simulink library "BatteryPack_v2"  (R2024b)
settings: Solver=VariableStepAuto  StartTime=0.0  StopTime=10.0  RelTol=1e-3
undefined symbols (not defined in the file or in its folder): battery_builder_rtmsupport, gcbh
libraries: BatteryPack_v2_lib x161
(part 6 of 8)

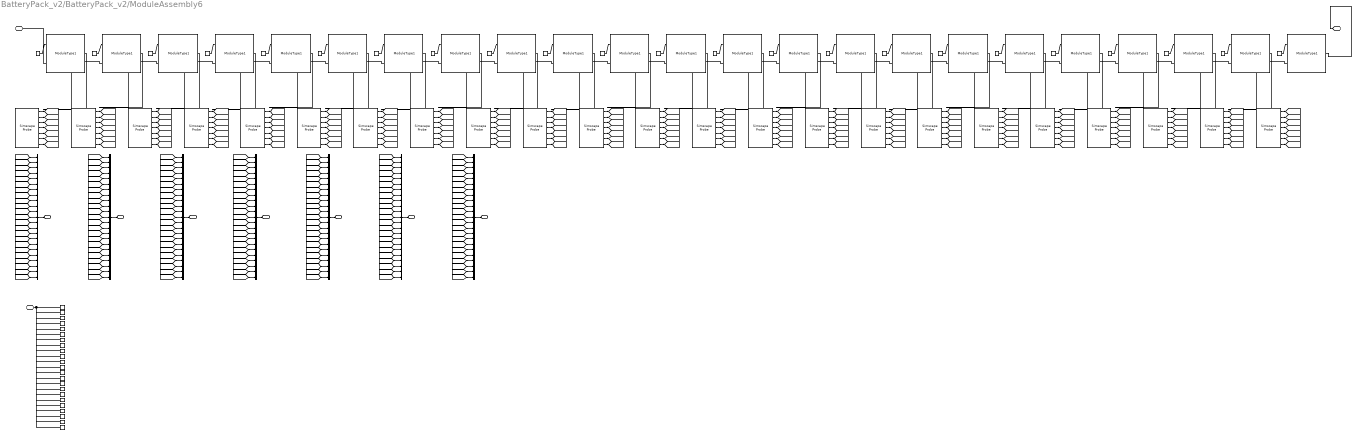
== system BatteryPack_v2/BatteryPack_v2/ModuleAssembly6 ==
  note: Thermal Boundary Conditions
  note: Output Signals
  note: Battery Modules
  AmbH_From_1 : ConnectionLabel  Label=ambH_1
  AmbH_From_10 : ConnectionLabel  Label=ambH_10
  AmbH_From_11 : ConnectionLabel  Label=ambH_11
  AmbH_From_12 : ConnectionLabel  Label=ambH_12
  AmbH_From_13 : ConnectionLabel  Label=ambH_13
  AmbH_From_14 : ConnectionLabel  Label=ambH_14
  AmbH_From_15 : ConnectionLabel  Label=ambH_15
  AmbH_From_16 : ConnectionLabel  Label=ambH_16
  AmbH_From_17 : ConnectionLabel  Label=ambH_17
  AmbH_From_18 : ConnectionLabel  Label=ambH_18
  AmbH_From_19 : ConnectionLabel  Label=ambH_19
  AmbH_From_2 : ConnectionLabel  Label=ambH_2
  AmbH_From_20 : ConnectionLabel  Label=ambH_20
  AmbH_From_21 : ConnectionLabel  Label=ambH_21
  AmbH_From_22 : ConnectionLabel  Label=ambH_22
  AmbH_From_23 : ConnectionLabel  Label=ambH_23
  AmbH_From_3 : ConnectionLabel  Label=ambH_3
  AmbH_From_4 : ConnectionLabel  Label=ambH_4
  AmbH_From_5 : ConnectionLabel  Label=ambH_5
  AmbH_From_6 : ConnectionLabel  Label=ambH_6
  AmbH_From_7 : ConnectionLabel  Label=ambH_7
  AmbH_From_8 : ConnectionLabel  Label=ambH_8
  AmbH_From_9 : ConnectionLabel  Label=ambH_9
  AmbH_To_1 : ConnectionLabel  Label=ambH_1
  AmbH_To_10 : ConnectionLabel  Label=ambH_10
  AmbH_To_11 : ConnectionLabel  Label=ambH_11
  AmbH_To_12 : ConnectionLabel  Label=ambH_12
  AmbH_To_13 : ConnectionLabel  Label=ambH_13
  AmbH_To_14 : ConnectionLabel  Label=ambH_14
  AmbH_To_15 : ConnectionLabel  Label=ambH_15
  AmbH_To_16 : ConnectionLabel  Label=ambH_16
  AmbH_To_17 : ConnectionLabel  Label=ambH_17
  AmbH_To_18 : ConnectionLabel  Label=ambH_18
  AmbH_To_19 : ConnectionLabel  Label=ambH_19
  AmbH_To_2 : ConnectionLabel  Label=ambH_2
  AmbH_To_20 : ConnectionLabel  Label=ambH_20
  AmbH_To_21 : ConnectionLabel  Label=ambH_21
  AmbH_To_22 : ConnectionLabel  Label=ambH_22
  AmbH_To_23 : ConnectionLabel  Label=ambH_23
  AmbH_To_3 : ConnectionLabel  Label=ambH_3
  AmbH_To_4 : ConnectionLabel  Label=ambH_4
  AmbH_To_5 : ConnectionLabel  Label=ambH_5
  AmbH_To_6 : ConnectionLabel  Label=ambH_6
  AmbH_To_7 : ConnectionLabel  Label=ambH_7
  AmbH_To_8 : ConnectionLabel  Label=ambH_8
  AmbH_To_9 : ConnectionLabel  Label=ambH_9
  Module02 : BatteryPack_v2_lib/Modules/ModuleType1  SOC_vecCell=[0, .1, .25, .5, .75, .9, 1]  T_vecCell=[278, 293, 313] K  V0_matCell=[3.49, 3.5, 3.51; 3.55, 3.57, 3.56; 3.62, 3.63, 3.64; 3.71, 3.71, 3.72; 3.91, 3.93, 3.94; 4.07, 4.08, 4.08; 4.19, 4.19, 4.19] V  V_rangeCell=[0, inf] V  R0_matCell=[.0117, .0085, .009; .011, .0085, .009; .0114, .0087, .0092; .0107, .0082, .0088; .0107, .0083, .0091; .0113, .0085, .0089; .0116, .0085, .0089] Ohm  AHCell=27 A*hr  extrapolation_optionCell=simscape.enum.extrapolation.nearest  N0Cell=100  dV0Cell=0  dR0Cell=0  dAHCell=0  thermal_massCell=100 J/K  AmbientResistance=25 K/W  P=1  S=1  iCell_specify=off  iCell_priority=None  iCell=0 A  iCell_nominal_specify=off  iCell_nominal_value=1  iCell_nominal_unit=A  vCell_specify=off  vCell_priority=None  vCell=0 V  vCell_nominal_specify=off  vCell_nominal_value=1  vCell_nominal_unit=V  socCell_specify=off  socCell_priority=High  socCell=1  socCell_nominal_specify=off  socCell_nominal_value=1  socCell_nominal_unit=1  numCyclesCell_specify=off  numCyclesCell_priority=High  numCyclesCell=0  numCyclesCell_nominal_specify=off  numCyclesCell_nominal_value=1  numCyclesCell_nominal_unit=1  temperatureCell_specify=off  temperatureCell_priority=High  temperatureCell=298.15 K  temperatureCell_nominal_specify=off  temperatureCell_nominal_value=1  temperatureCell_nominal_unit=K  vParallelAssembly_specify=off  vParallelAssembly_priority=None  vParallelAssembly=0 V  vParallelAssembly_nominal_specify=off  vParallelAssembly_nominal_value=1  vParallelAssembly_nominal_unit=V  socParallelAssembly_specify=off  socParallelAssembly_priority=None  socParallelAssembly=1  socParallelAssembly_nominal_specify=off  socParallelAssembly_nominal_value=1  socParallelAssembly_nominal_unit=1
      settings: InternalSimscapePortConfiguration="{\"Bottom\":[{\"id\":\"n\",\"label\":\"-\",\"type\":\"foundation.electrical.electrical\"}],\"Left\":[{\"id\":\"AmbH\",\"label\":\"AmbH\",\"type\":\"foundation.thermal.thermal\"}],\"Right\":[],\"Top\":[{\"id\":\"p\",\"label\":\"+\",\"type\":\"foundation.electrical.electrical\"}]}"
  Module02_outputs : SimscapeProbe  BoundBlock=2660  Variables="{\"iCell\":{\"Unit\":\"A\",\"PortLabel\":\"iCell\",\"Probing\":\"ON\"},\"numCyclesCell\":{\"Unit\":\"1\",\"PortLabel\":\"numCyclesCell\",\"Probing\":\"ON\"},\"socCell\":{\"Unit\":\"1\",\"PortLabel\":\"socCell\",\"Probing\":\"ON\"},\"socParallelAssembly\":{\"Unit\":\"1\",\"PortLabel\":\"socParallelAssembly\",\"Probing\":\"ON\"},\"temperatureCell\":{\"Unit\":\"K\",\"PortLabel\":\"temperatureCell\",\"Probing\":\"ON\"},\"vCell\":{\"Unit\":\"V\",\"PortLabel\":\"vCell\",\"Probing\":\"ON\"},\"vParallelAssembly\":{\"Unit\":\"V\",\"PortLabel\":\"vParallelAssembly\",\"Probing\":\"ON\"}}"
  Module03 : BatteryPack_v2_lib/Modules/ModuleType1  SOC_vecCell=[0, .1, .25, .5, .75, .9, 1]  T_vecCell=[278, 293, 313] K  V0_matCell=[3.49, 3.5, 3.51; 3.55, 3.57, 3.56; 3.62, 3.63, 3.64; 3.71, 3.71, 3.72; 3.91, 3.93, 3.94; 4.07, 4.08, 4.08; 4.19, 4.19, 4.19] V  V_rangeCell=[0, inf] V  R0_matCell=[.0117, .0085, .009; .011, .0085, .009; .0114, .0087, .0092; .0107, .0082, .0088; .0107, .0083, .0091; .0113, .0085, .0089; .0116, .0085, .0089] Ohm  AHCell=27 A*hr  extrapolation_optionCell=simscape.enum.extrapolation.nearest  N0Cell=100  dV0Cell=0  dR0Cell=0  dAHCell=0  thermal_massCell=100 J/K  AmbientResistance=25 K/W  P=1  S=1  iCell_specify=off  iCell_priority=None  iCell=0 A  iCell_nominal_specify=off  iCell_nominal_value=1  iCell_nominal_unit=A  vCell_specify=off  vCell_priority=None  vCell=0 V  vCell_nominal_specify=off  vCell_nominal_value=1  vCell_nominal_unit=V  socCell_specify=off  socCell_priority=High  socCell=1  socCell_nominal_specify=off  socCell_nominal_value=1  socCell_nominal_unit=1  numCyclesCell_specify=off  numCyclesCell_priority=High  numCyclesCell=0  numCyclesCell_nominal_specify=off  numCyclesCell_nominal_value=1  numCyclesCell_nominal_unit=1  temperatureCell_specify=off  temperatureCell_priority=High  temperatureCell=298.15 K  temperatureCell_nominal_specify=off  temperatureCell_nominal_value=1  temperatureCell_nominal_unit=K  vParallelAssembly_specify=off  vParallelAssembly_priority=None  vParallelAssembly=0 V  vParallelAssembly_nominal_specify=off  vParallelAssembly_nominal_value=1  vParallelAssembly_nominal_unit=V  socParallelAssembly_specify=off  socParallelAssembly_priority=None  socParallelAssembly=1  socParallelAssembly_nominal_specify=off  socParallelAssembly_nominal_value=1  socParallelAssembly_nominal_unit=1
      settings: InternalSimscapePortConfiguration="{\"Bottom\":[{\"id\":\"n\",\"label\":\"-\",\"type\":\"foundation.electrical.electrical\"}],\"Left\":[{\"id\":\"AmbH\",\"label\":\"AmbH\",\"type\":\"foundation.thermal.thermal\"}],\"Right\":[],\"Top\":[{\"id\":\"p\",\"label\":\"+\",\"type\":\"foundation.electrical.electrical\"}]}"
  Module03_outputs : SimscapeProbe  BoundBlock=2662  Variables="{\"iCell\":{\"Unit\":\"A\",\"PortLabel\":\"iCell\",\"Probing\":\"ON\"},\"numCyclesCell\":{\"Unit\":\"1\",\"PortLabel\":\"numCyclesCell\",\"Probing\":\"ON\"},\"socCell\":{\"Unit\":\"1\",\"PortLabel\":\"socCell\",\"Probing\":\"ON\"},\"socParallelAssembly\":{\"Unit\":\"1\",\"PortLabel\":\"socParallelAssembly\",\"Probing\":\"ON\"},\"temperatureCell\":{\"Unit\":\"K\",\"PortLabel\":\"temperatureCell\",\"Probing\":\"ON\"},\"vCell\":{\"Unit\":\"V\",\"PortLabel\":\"vCell\",\"Probing\":\"ON\"},\"vParallelAssembly\":{\"Unit\":\"V\",\"PortLabel\":\"vParallelAssembly\",\"Probing\":\"ON\"}}"
  Module04 : BatteryPack_v2_lib/Modules/ModuleType1  SOC_vecCell=[0, .1, .25, .5, .75, .9, 1]  T_vecCell=[278, 293, 313] K  V0_matCell=[3.49, 3.5, 3.51; 3.55, 3.57, 3.56; 3.62, 3.63, 3.64; 3.71, 3.71, 3.72; 3.91, 3.93, 3.94; 4.07, 4.08, 4.08; 4.19, 4.19, 4.19] V  V_rangeCell=[0, inf] V  R0_matCell=[.0117, .0085, .009; .011, .0085, .009; .0114, .0087, .0092; .0107, .0082, .0088; .0107, .0083, .0091; .0113, .0085, .0089; .0116, .0085, .0089] Ohm  AHCell=27 A*hr  extrapolation_optionCell=simscape.enum.extrapolation.nearest  N0Cell=100  dV0Cell=0  dR0Cell=0  dAHCell=0  thermal_massCell=100 J/K  AmbientResistance=25 K/W  P=1  S=1  iCell_specify=off  iCell_priority=None  iCell=0 A  iCell_nominal_specify=off  iCell_nominal_value=1  iCell_nominal_unit=A  vCell_specify=off  vCell_priority=None  vCell=0 V  vCell_nominal_specify=off  vCell_nominal_value=1  vCell_nominal_unit=V  socCell_specify=off  socCell_priority=High  socCell=1  socCell_nominal_specify=off  socCell_nominal_value=1  socCell_nominal_unit=1  numCyclesCell_specify=off  numCyclesCell_priority=High  numCyclesCell=0  numCyclesCell_nominal_specify=off  numCyclesCell_nominal_value=1  numCyclesCell_nominal_unit=1  temperatureCell_specify=off  temperatureCell_priority=High  temperatureCell=298.15 K  temperatureCell_nominal_specify=off  temperatureCell_nominal_value=1  temperatureCell_nominal_unit=K  vParallelAssembly_specify=off  vParallelAssembly_priority=None  vParallelAssembly=0 V  vParallelAssembly_nominal_specify=off  vParallelAssembly_nominal_value=1  vParallelAssembly_nominal_unit=V  socParallelAssembly_specify=off  socParallelAssembly_priority=None  socParallelAssembly=1  socParallelAssembly_nominal_specify=off  socParallelAssembly_nominal_value=1  socParallelAssembly_nominal_unit=1
      settings: InternalSimscapePortConfiguration="{\"Bottom\":[{\"id\":\"n\",\"label\":\"-\",\"type\":\"foundation.electrical.electrical\"}],\"Left\":[{\"id\":\"AmbH\",\"label\":\"AmbH\",\"type\":\"foundation.thermal.thermal\"}],\"Right\":[],\"Top\":[{\"id\":\"p\",\"label\":\"+\",\"type\":\"foundation.electrical.electrical\"}]}"
  Module04_outputs : SimscapeProbe  BoundBlock=2664  Variables="{\"iCell\":{\"Unit\":\"A\",\"PortLabel\":\"iCell\",\"Probing\":\"ON\"},\"numCyclesCell\":{\"Unit\":\"1\",\"PortLabel\":\"numCyclesCell\",\"Probing\":\"ON\"},\"socCell\":{\"Unit\":\"1\",\"PortLabel\":\"socCell\",\"Probing\":\"ON\"},\"socParallelAssembly\":{\"Unit\":\"1\",\"PortLabel\":\"socParallelAssembly\",\"Probing\":\"ON\"},\"temperatureCell\":{\"Unit\":\"K\",\"PortLabel\":\"temperatureCell\",\"Probing\":\"ON\"},\"vCell\":{\"Unit\":\"V\",\"PortLabel\":\"vCell\",\"Probing\":\"ON\"},\"vParallelAssembly\":{\"Unit\":\"V\",\"PortLabel\":\"vParallelAssembly\",\"Probing\":\"ON\"}}"
  Module05 : BatteryPack_v2_lib/Modules/ModuleType1  SOC_vecCell=[0, .1, .25, .5, .75, .9, 1]  T_vecCell=[278, 293, 313] K  V0_matCell=[3.49, 3.5, 3.51; 3.55, 3.57, 3.56; 3.62, 3.63, 3.64; 3.71, 3.71, 3.72; 3.91, 3.93, 3.94; 4.07, 4.08, 4.08; 4.19, 4.19, 4.19] V  V_rangeCell=[0, inf] V  R0_matCell=[.0117, .0085, .009; .011, .0085, .009; .0114, .0087, .0092; .0107, .0082, .0088; .0107, .0083, .0091; .0113, .0085, .0089; .0116, .0085, .0089] Ohm  AHCell=27 A*hr  extrapolation_optionCell=simscape.enum.extrapolation.nearest  N0Cell=100  dV0Cell=0  dR0Cell=0  dAHCell=0  thermal_massCell=100 J/K  AmbientResistance=25 K/W  P=1  S=1  iCell_specify=off  iCell_priority=None  iCell=0 A  iCell_nominal_specify=off  iCell_nominal_value=1  iCell_nominal_unit=A  vCell_specify=off  vCell_priority=None  vCell=0 V  vCell_nominal_specify=off  vCell_nominal_value=1  vCell_nominal_unit=V  socCell_specify=off  socCell_priority=High  socCell=1  socCell_nominal_specify=off  socCell_nominal_value=1  socCell_nominal_unit=1  numCyclesCell_specify=off  numCyclesCell_priority=High  numCyclesCell=0  numCyclesCell_nominal_specify=off  numCyclesCell_nominal_value=1  numCyclesCell_nominal_unit=1  temperatureCell_specify=off  temperatureCell_priority=High  temperatureCell=298.15 K  temperatureCell_nominal_specify=off  temperatureCell_nominal_value=1  temperatureCell_nominal_unit=K  vParallelAssembly_specify=off  vParallelAssembly_priority=None  vParallelAssembly=0 V  vParallelAssembly_nominal_specify=off  vParallelAssembly_nominal_value=1  vParallelAssembly_nominal_unit=V  socParallelAssembly_specify=off  socParallelAssembly_priority=None  socParallelAssembly=1  socParallelAssembly_nominal_specify=off  socParallelAssembly_nominal_value=1  socParallelAssembly_nominal_unit=1
      settings: InternalSimscapePortConfiguration="{\"Bottom\":[{\"id\":\"n\",\"label\":\"-\",\"type\":\"foundation.electrical.electrical\"}],\"Left\":[{\"id\":\"AmbH\",\"label\":\"AmbH\",\"type\":\"foundation.thermal.thermal\"}],\"Right\":[],\"Top\":[{\"id\":\"p\",\"label\":\"+\",\"type\":\"foundation.electrical.electrical\"}]}"
  Module05_outputs : SimscapeProbe  BoundBlock=2666  Variables="{\"iCell\":{\"Unit\":\"A\",\"PortLabel\":\"iCell\",\"Probing\":\"ON\"},\"numCyclesCell\":{\"Unit\":\"1\",\"PortLabel\":\"numCyclesCell\",\"Probing\":\"ON\"},\"socCell\":{\"Unit\":\"1\",\"PortLabel\":\"socCell\",\"Probing\":\"ON\"},\"socParallelAssembly\":{\"Unit\":\"1\",\"PortLabel\":\"socParallelAssembly\",\"Probing\":\"ON\"},\"temperatureCell\":{\"Unit\":\"K\",\"PortLabel\":\"temperatureCell\",\"Probing\":\"ON\"},\"vCell\":{\"Unit\":\"V\",\"PortLabel\":\"vCell\",\"Probing\":\"ON\"},\"vParallelAssembly\":{\"Unit\":\"V\",\"PortLabel\":\"vParallelAssembly\",\"Probing\":\"ON\"}}"
  Module06 : BatteryPack_v2_lib/Modules/ModuleType1  SOC_vecCell=[0, .1, .25, .5, .75, .9, 1]  T_vecCell=[278, 293, 313] K  V0_matCell=[3.49, 3.5, 3.51; 3.55, 3.57, 3.56; 3.62, 3.63, 3.64; 3.71, 3.71, 3.72; 3.91, 3.93, 3.94; 4.07, 4.08, 4.08; 4.19, 4.19, 4.19] V  V_rangeCell=[0, inf] V  R0_matCell=[.0117, .0085, .009; .011, .0085, .009; .0114, .0087, .0092; .0107, .0082, .0088; .0107, .0083, .0091; .0113, .0085, .0089; .0116, .0085, .0089] Ohm  AHCell=27 A*hr  extrapolation_optionCell=simscape.enum.extrapolation.nearest  N0Cell=100  dV0Cell=0  dR0Cell=0  dAHCell=0  thermal_massCell=100 J/K  AmbientResistance=25 K/W  P=1  S=1  iCell_specify=off  iCell_priority=None  iCell=0 A  iCell_nominal_specify=off  iCell_nominal_value=1  iCell_nominal_unit=A  vCell_specify=off  vCell_priority=None  vCell=0 V  vCell_nominal_specify=off  vCell_nominal_value=1  vCell_nominal_unit=V  socCell_specify=off  socCell_priority=High  socCell=1  socCell_nominal_specify=off  socCell_nominal_value=1  socCell_nominal_unit=1  numCyclesCell_specify=off  numCyclesCell_priority=High  numCyclesCell=0  numCyclesCell_nominal_specify=off  numCyclesCell_nominal_value=1  numCyclesCell_nominal_unit=1  temperatureCell_specify=off  temperatureCell_priority=High  temperatureCell=298.15 K  temperatureCell_nominal_specify=off  temperatureCell_nominal_value=1  temperatureCell_nominal_unit=K  vParallelAssembly_specify=off  vParallelAssembly_priority=None  vParallelAssembly=0 V  vParallelAssembly_nominal_specify=off  vParallelAssembly_nominal_value=1  vParallelAssembly_nominal_unit=V  socParallelAssembly_specify=off  socParallelAssembly_priority=None  socParallelAssembly=1  socParallelAssembly_nominal_specify=off  socParallelAssembly_nominal_value=1  socParallelAssembly_nominal_unit=1
      settings: InternalSimscapePortConfiguration="{\"Bottom\":[{\"id\":\"n\",\"label\":\"-\",\"type\":\"foundation.electrical.electrical\"}],\"Left\":[{\"id\":\"AmbH\",\"label\":\"AmbH\",\"type\":\"foundation.thermal.thermal\"}],\"Right\":[],\"Top\":[{\"id\":\"p\",\"label\":\"+\",\"type\":\"foundation.electrical.electrical\"}]}"
  Module06_outputs : SimscapeProbe  BoundBlock=2668  Variables="{\"iCell\":{\"Unit\":\"A\",\"PortLabel\":\"iCell\",\"Probing\":\"ON\"},\"numCyclesCell\":{\"Unit\":\"1\",\"PortLabel\":\"numCyclesCell\",\"Probing\":\"ON\"},\"socCell\":{\"Unit\":\"1\",\"PortLabel\":\"socCell\",\"Probing\":\"ON\"},\"socParallelAssembly\":{\"Unit\":\"1\",\"PortLabel\":\"socParallelAssembly\",\"Probing\":\"ON\"},\"temperatureCell\":{\"Unit\":\"K\",\"PortLabel\":\"temperatureCell\",\"Probing\":\"ON\"},\"vCell\":{\"Unit\":\"V\",\"PortLabel\":\"vCell\",\"Probing\":\"ON\"},\"vParallelAssembly\":{\"Unit\":\"V\",\"PortLabel\":\"vParallelAssembly\",\"Probing\":\"ON\"}}"
  Module07 : BatteryPack_v2_lib/Modules/ModuleType1  SOC_vecCell=[0, .1, .25, .5, .75, .9, 1]  T_vecCell=[278, 293, 313] K  V0_matCell=[3.49, 3.5, 3.51; 3.55, 3.57, 3.56; 3.62, 3.63, 3.64; 3.71, 3.71, 3.72; 3.91, 3.93, 3.94; 4.07, 4.08, 4.08; 4.19, 4.19, 4.19] V  V_rangeCell=[0, inf] V  R0_matCell=[.0117, .0085, .009; .011, .0085, .009; .0114, .0087, .0092; .0107, .0082, .0088; .0107, .0083, .0091; .0113, .0085, .0089; .0116, .0085, .0089] Ohm  AHCell=27 A*hr  extrapolation_optionCell=simscape.enum.extrapolation.nearest  N0Cell=100  dV0Cell=0  dR0Cell=0  dAHCell=0  thermal_massCell=100 J/K  AmbientResistance=25 K/W  P=1  S=1  iCell_specify=off  iCell_priority=None  iCell=0 A  iCell_nominal_specify=off  iCell_nominal_value=1  iCell_nominal_unit=A  vCell_specify=off  vCell_priority=None  vCell=0 V  vCell_nominal_specify=off  vCell_nominal_value=1  vCell_nominal_unit=V  socCell_specify=off  socCell_priority=High  socCell=1  socCell_nominal_specify=off  socCell_nominal_value=1  socCell_nominal_unit=1  numCyclesCell_specify=off  numCyclesCell_priority=High  numCyclesCell=0  numCyclesCell_nominal_specify=off  numCyclesCell_nominal_value=1  numCyclesCell_nominal_unit=1  temperatureCell_specify=off  temperatureCell_priority=High  temperatureCell=298.15 K  temperatureCell_nominal_specify=off  temperatureCell_nominal_value=1  temperatureCell_nominal_unit=K  vParallelAssembly_specify=off  vParallelAssembly_priority=None  vParallelAssembly=0 V  vParallelAssembly_nominal_specify=off  vParallelAssembly_nominal_value=1  vParallelAssembly_nominal_unit=V  socParallelAssembly_specify=off  socParallelAssembly_priority=None  socParallelAssembly=1  socParallelAssembly_nominal_specify=off  socParallelAssembly_nominal_value=1  socParallelAssembly_nominal_unit=1
      settings: InternalSimscapePortConfiguration="{\"Bottom\":[{\"id\":\"n\",\"label\":\"-\",\"type\":\"foundation.electrical.electrical\"}],\"Left\":[{\"id\":\"AmbH\",\"label\":\"AmbH\",\"type\":\"foundation.thermal.thermal\"}],\"Right\":[],\"Top\":[{\"id\":\"p\",\"label\":\"+\",\"type\":\"foundation.electrical.electrical\"}]}"
  Module07_outputs : SimscapeProbe  BoundBlock=2670  Variables="{\"iCell\":{\"Unit\":\"A\",\"PortLabel\":\"iCell\",\"Probing\":\"ON\"},\"numCyclesCell\":{\"Unit\":\"1\",\"PortLabel\":\"numCyclesCell\",\"Probing\":\"ON\"},\"socCell\":{\"Unit\":\"1\",\"PortLabel\":\"socCell\",\"Probing\":\"ON\"},\"socParallelAssembly\":{\"Unit\":\"1\",\"PortLabel\":\"socParallelAssembly\",\"Probing\":\"ON\"},\"temperatureCell\":{\"Unit\":\"K\",\"PortLabel\":\"temperatureCell\",\"Probing\":\"ON\"},\"vCell\":{\"Unit\":\"V\",\"PortLabel\":\"vCell\",\"Probing\":\"ON\"},\"vParallelAssembly\":{\"Unit\":\"V\",\"PortLabel\":\"vParallelAssembly\",\"Probing\":\"ON\"}}"
  Module08 : BatteryPack_v2_lib/Modules/ModuleType1  SOC_vecCell=[0, .1, .25, .5, .75, .9, 1]  T_vecCell=[278, 293, 313] K  V0_matCell=[3.49, 3.5, 3.51; 3.55, 3.57, 3.56; 3.62, 3.63, 3.64; 3.71, 3.71, 3.72; 3.91, 3.93, 3.94; 4.07, 4.08, 4.08; 4.19, 4.19, 4.19] V  V_rangeCell=[0, inf] V  R0_matCell=[.0117, .0085, .009; .011, .0085, .009; .0114, .0087, .0092; .0107, .0082, .0088; .0107, .0083, .0091; .0113, .0085, .0089; .0116, .0085, .0089] Ohm  AHCell=27 A*hr  extrapolation_optionCell=simscape.enum.extrapolation.nearest  N0Cell=100  dV0Cell=0  dR0Cell=0  dAHCell=0  thermal_massCell=100 J/K  AmbientResistance=25 K/W  P=1  S=1  iCell_specify=off  iCell_priority=None  iCell=0 A  iCell_nominal_specify=off  iCell_nominal_value=1  iCell_nominal_unit=A  vCell_specify=off  vCell_priority=None  vCell=0 V  vCell_nominal_specify=off  vCell_nominal_value=1  vCell_nominal_unit=V  socCell_specify=off  socCell_priority=High  socCell=1  socCell_nominal_specify=off  socCell_nominal_value=1  socCell_nominal_unit=1  numCyclesCell_specify=off  numCyclesCell_priority=High  numCyclesCell=0  numCyclesCell_nominal_specify=off  numCyclesCell_nominal_value=1  numCyclesCell_nominal_unit=1  temperatureCell_specify=off  temperatureCell_priority=High  temperatureCell=298.15 K  temperatureCell_nominal_specify=off  temperatureCell_nominal_value=1  temperatureCell_nominal_unit=K  vParallelAssembly_specify=off  vParallelAssembly_priority=None  vParallelAssembly=0 V  vParallelAssembly_nominal_specify=off  vParallelAssembly_nominal_value=1  vParallelAssembly_nominal_unit=V  socParallelAssembly_specify=off  socParallelAssembly_priority=None  socParallelAssembly=1  socParallelAssembly_nominal_specify=off  socParallelAssembly_nominal_value=1  socParallelAssembly_nominal_unit=1
      settings: InternalSimscapePortConfiguration="{\"Bottom\":[{\"id\":\"n\",\"label\":\"-\",\"type\":\"foundation.electrical.electrical\"}],\"Left\":[{\"id\":\"AmbH\",\"label\":\"AmbH\",\"type\":\"foundation.thermal.thermal\"}],\"Right\":[],\"Top\":[{\"id\":\"p\",\"label\":\"+\",\"type\":\"foundation.electrical.electrical\"}]}"
  Module08_outputs : SimscapeProbe  BoundBlock=2672  Variables="{\"iCell\":{\"Unit\":\"A\",\"PortLabel\":\"iCell\",\"Probing\":\"ON\"},\"numCyclesCell\":{\"Unit\":\"1\",\"PortLabel\":\"numCyclesCell\",\"Probing\":\"ON\"},\"socCell\":{\"Unit\":\"1\",\"PortLabel\":\"socCell\",\"Probing\":\"ON\"},\"socParallelAssembly\":{\"Unit\":\"1\",\"PortLabel\":\"socParallelAssembly\",\"Probing\":\"ON\"},\"temperatureCell\":{\"Unit\":\"K\",\"PortLabel\":\"temperatureCell\",\"Probing\":\"ON\"},\"vCell\":{\"Unit\":\"V\",\"PortLabel\":\"vCell\",\"Probing\":\"ON\"},\"vParallelAssembly\":{\"Unit\":\"V\",\"PortLabel\":\"vParallelAssembly\",\"Probing\":\"ON\"}}"
  Module09 : BatteryPack_v2_lib/Modules/ModuleType1  SOC_vecCell=[0, .1, .25, .5, .75, .9, 1]  T_vecCell=[278, 293, 313] K  V0_matCell=[3.49, 3.5, 3.51; 3.55, 3.57, 3.56; 3.62, 3.63, 3.64; 3.71, 3.71, 3.72; 3.91, 3.93, 3.94; 4.07, 4.08, 4.08; 4.19, 4.19, 4.19] V  V_rangeCell=[0, inf] V  R0_matCell=[.0117, .0085, .009; .011, .0085, .009; .0114, .0087, .0092; .0107, .0082, .0088; .0107, .0083, .0091; .0113, .0085, .0089; .0116, .0085, .0089] Ohm  AHCell=27 A*hr  extrapolation_optionCell=simscape.enum.extrapolation.nearest  N0Cell=100  dV0Cell=0  dR0Cell=0  dAHCell=0  thermal_massCell=100 J/K  AmbientResistance=25 K/W  P=1  S=1  iCell_specify=off  iCell_priority=None  iCell=0 A  iCell_nominal_specify=off  iCell_nominal_value=1  iCell_nominal_unit=A  vCell_specify=off  vCell_priority=None  vCell=0 V  vCell_nominal_specify=off  vCell_nominal_value=1  vCell_nominal_unit=V  socCell_specify=off  socCell_priority=High  socCell=1  socCell_nominal_specify=off  socCell_nominal_value=1  socCell_nominal_unit=1  numCyclesCell_specify=off  numCyclesCell_priority=High  numCyclesCell=0  numCyclesCell_nominal_specify=off  numCyclesCell_nominal_value=1  numCyclesCell_nominal_unit=1  temperatureCell_specify=off  temperatureCell_priority=High  temperatureCell=298.15 K  temperatureCell_nominal_specify=off  temperatureCell_nominal_value=1  temperatureCell_nominal_unit=K  vParallelAssembly_specify=off  vParallelAssembly_priority=None  vParallelAssembly=0 V  vParallelAssembly_nominal_specify=off  vParallelAssembly_nominal_value=1  vParallelAssembly_nominal_unit=V  socParallelAssembly_specify=off  socParallelAssembly_priority=None  socParallelAssembly=1  socParallelAssembly_nominal_specify=off  socParallelAssembly_nominal_value=1  socParallelAssembly_nominal_unit=1
      settings: InternalSimscapePortConfiguration="{\"Bottom\":[{\"id\":\"n\",\"label\":\"-\",\"type\":\"foundation.electrical.electrical\"}],\"Left\":[{\"id\":\"AmbH\",\"label\":\"AmbH\",\"type\":\"foundation.thermal.thermal\"}],\"Right\":[],\"Top\":[{\"id\":\"p\",\"label\":\"+\",\"type\":\"foundation.electrical.electrical\"}]}"
  Module09_outputs : SimscapeProbe  BoundBlock=2674  Variables="{\"iCell\":{\"Unit\":\"A\",\"PortLabel\":\"iCell\",\"Probing\":\"ON\"},\"numCyclesCell\":{\"Unit\":\"1\",\"PortLabel\":\"numCyclesCell\",\"Probing\":\"ON\"},\"socCell\":{\"Unit\":\"1\",\"PortLabel\":\"socCell\",\"Probing\":\"ON\"},\"socParallelAssembly\":{\"Unit\":\"1\",\"PortLabel\":\"socParallelAssembly\",\"Probing\":\"ON\"},\"temperatureCell\":{\"Unit\":\"K\",\"PortLabel\":\"temperatureCell\",\"Probing\":\"ON\"},\"vCell\":{\"Unit\":\"V\",\"PortLabel\":\"vCell\",\"Probing\":\"ON\"},\"vParallelAssembly\":{\"Unit\":\"V\",\"PortLabel\":\"vParallelAssembly\",\"Probing\":\"ON\"}}"
  Module{10..23} (14 alike) : BatteryPack_v2_lib/Modules/ModuleType1  SOC_vecCell=[0, .1, .25, .5, .75, .9, 1]  T_vecCell=[278, 293, 313] K  V0_matCell=[3.49, 3.5, 3.51; 3.55, 3.57, 3.56; 3.62, 3.63, 3.64; 3.71, 3.71, 3.72; 3.91, 3.93, 3.94; 4.07, 4.08, 4.08; 4.19, 4.19, 4.19] V  V_rangeCell=[0, inf] V  R0_matCell=[.0117, .0085, .009; .011, .0085, .009; .0114, .0087, .0092; .0107, .0082, .0088; .0107, .0083, .0091; .0113, .0085, .0089; .0116, .0085, .0089] Ohm  AHCell=27 A*hr  extrapolation_optionCell=simscape.enum.extrapolation.nearest  N0Cell=100  dV0Cell=0  dR0Cell=0  dAHCell=0  thermal_massCell=100 J/K  AmbientResistance=25 K/W  P=1  S=1  iCell_specify=off  iCell_priority=None  iCell=0 A  iCell_nominal_specify=off  iCell_nominal_value=1  iCell_nominal_unit=A  vCell_specify=off  vCell_priority=None  vCell=0 V  vCell_nominal_specify=off  vCell_nominal_value=1  vCell_nominal_unit=V  socCell_specify=off  socCell_priority=High  socCell=1  socCell_nominal_specify=off  socCell_nominal_value=1  socCell_nominal_unit=1  numCyclesCell_specify=off  numCyclesCell_priority=High  numCyclesCell=0  numCyclesCell_nominal_specify=off  numCyclesCell_nominal_value=1  numCyclesCell_nominal_unit=1  temperatureCell_specify=off  temperatureCell_priority=High  temperatureCell=298.15 K  temperatureCell_nominal_specify=off  temperatureCell_nominal_value=1  temperatureCell_nominal_unit=K  vParallelAssembly_specify=off  vParallelAssembly_priority=None  vParallelAssembly=0 V  vParallelAssembly_nominal_specify=off  vParallelAssembly_nominal_value=1  vParallelAssembly_nominal_unit=V  socParallelAssembly_specify=off  socParallelAssembly_priority=None  socParallelAssembly=1  socParallelAssembly_nominal_specify=off  socParallelAssembly_nominal_value=1  socParallelAssembly_nominal_unit=1
      settings: InternalSimscapePortConfiguration="{\"Bottom\":[{\"id\":\"n\",\"label\":\"-\",\"type\":\"foundation.electrical.electrical\"}],\"Left\":[{\"id\":\"AmbH\",\"label\":\"AmbH\",\"type\":\"foundation.thermal.thermal\"}],\"Right\":[],\"Top\":[{\"id\":\"p\",\"label\":\"+\",\"type\":\"foundation.electrical.electrical\"}]}"
  Module10_outputs : SimscapeProbe  BoundBlock=2676  Variables="{\"iCell\":{\"Unit\":\"A\",\"PortLabel\":\"iCell\",\"Probing\":\"ON\"},\"numCyclesCell\":{\"Unit\":\"1\",\"PortLabel\":\"numCyclesCell\",\"Probing\":\"ON\"},\"socCell\":{\"Unit\":\"1\",\"PortLabel\":\"socCell\",\"Probing\":\"ON\"},\"socParallelAssembly\":{\"Unit\":\"1\",\"PortLabel\":\"socParallelAssembly\",\"Probing\":\"ON\"},\"temperatureCell\":{\"Unit\":\"K\",\"PortLabel\":\"temperatureCell\",\"Probing\":\"ON\"},\"vCell\":{\"Unit\":\"V\",\"PortLabel\":\"vCell\",\"Probing\":\"ON\"},\"vParallelAssembly\":{\"Unit\":\"V\",\"PortLabel\":\"vParallelAssembly\",\"Probing\":\"ON\"}}"
  Module11_outputs : SimscapeProbe  BoundBlock=2678  Variables="{\"iCell\":{\"Unit\":\"A\",\"PortLabel\":\"iCell\",\"Probing\":\"ON\"},\"numCyclesCell\":{\"Unit\":\"1\",\"PortLabel\":\"numCyclesCell\",\"Probing\":\"ON\"},\"socCell\":{\"Unit\":\"1\",\"PortLabel\":\"socCell\",\"Probing\":\"ON\"},\"socParallelAssembly\":{\"Unit\":\"1\",\"PortLabel\":\"socParallelAssembly\",\"Probing\":\"ON\"},\"temperatureCell\":{\"Unit\":\"K\",\"PortLabel\":\"temperatureCell\",\"Probing\":\"ON\"},\"vCell\":{\"Unit\":\"V\",\"PortLabel\":\"vCell\",\"Probing\":\"ON\"},\"vParallelAssembly\":{\"Unit\":\"V\",\"PortLabel\":\"vParallelAssembly\",\"Probing\":\"ON\"}}"
  Module12_outputs : SimscapeProbe  BoundBlock=2680  Variables="{\"iCell\":{\"Unit\":\"A\",\"PortLabel\":\"iCell\",\"Probing\":\"ON\"},\"numCyclesCell\":{\"Unit\":\"1\",\"PortLabel\":\"numCyclesCell\",\"Probing\":\"ON\"},\"socCell\":{\"Unit\":\"1\",\"PortLabel\":\"socCell\",\"Probing\":\"ON\"},\"socParallelAssembly\":{\"Unit\":\"1\",\"PortLabel\":\"socParallelAssembly\",\"Probing\":\"ON\"},\"temperatureCell\":{\"Unit\":\"K\",\"PortLabel\":\"temperatureCell\",\"Probing\":\"ON\"},\"vCell\":{\"Unit\":\"V\",\"PortLabel\":\"vCell\",\"Probing\":\"ON\"},\"vParallelAssembly\":{\"Unit\":\"V\",\"PortLabel\":\"vParallelAssembly\",\"Probing\":\"ON\"}}"
  Module13_outputs : SimscapeProbe  BoundBlock=2682  Variables="{\"iCell\":{\"Unit\":\"A\",\"PortLabel\":\"iCell\",\"Probing\":\"ON\"},\"numCyclesCell\":{\"Unit\":\"1\",\"PortLabel\":\"numCyclesCell\",\"Probing\":\"ON\"},\"socCell\":{\"Unit\":\"1\",\"PortLabel\":\"socCell\",\"Probing\":\"ON\"},\"socParallelAssembly\":{\"Unit\":\"1\",\"PortLabel\":\"socParallelAssembly\",\"Probing\":\"ON\"},\"temperatureCell\":{\"Unit\":\"K\",\"PortLabel\":\"temperatureCell\",\"Probing\":\"ON\"},\"vCell\":{\"Unit\":\"V\",\"PortLabel\":\"vCell\",\"Probing\":\"ON\"},\"vParallelAssembly\":{\"Unit\":\"V\",\"PortLabel\":\"vParallelAssembly\",\"Probing\":\"ON\"}}"
  Module14_outputs : SimscapeProbe  BoundBlock=2684  Variables="{\"iCell\":{\"Unit\":\"A\",\"PortLabel\":\"iCell\",\"Probing\":\"ON\"},\"numCyclesCell\":{\"Unit\":\"1\",\"PortLabel\":\"numCyclesCell\",\"Probing\":\"ON\"},\"socCell\":{\"Unit\":\"1\",\"PortLabel\":\"socCell\",\"Probing\":\"ON\"},\"socParallelAssembly\":{\"Unit\":\"1\",\"PortLabel\":\"socParallelAssembly\",\"Probing\":\"ON\"},\"temperatureCell\":{\"Unit\":\"K\",\"PortLabel\":\"temperatureCell\",\"Probing\":\"ON\"},\"vCell\":{\"Unit\":\"V\",\"PortLabel\":\"vCell\",\"Probing\":\"ON\"},\"vParallelAssembly\":{\"Unit\":\"V\",\"PortLabel\":\"vParallelAssembly\",\"Probing\":\"ON\"}}"
  Module15_outputs : SimscapeProbe  BoundBlock=2686  Variables="{\"iCell\":{\"Unit\":\"A\",\"PortLabel\":\"iCell\",\"Probing\":\"ON\"},\"numCyclesCell\":{\"Unit\":\"1\",\"PortLabel\":\"numCyclesCell\",\"Probing\":\"ON\"},\"socCell\":{\"Unit\":\"1\",\"PortLabel\":\"socCell\",\"Probing\":\"ON\"},\"socParallelAssembly\":{\"Unit\":\"1\",\"PortLabel\":\"socParallelAssembly\",\"Probing\":\"ON\"},\"temperatureCell\":{\"Unit\":\"K\",\"PortLabel\":\"temperatureCell\",\"Probing\":\"ON\"},\"vCell\":{\"Unit\":\"V\",\"PortLabel\":\"vCell\",\"Probing\":\"ON\"},\"vParallelAssembly\":{\"Unit\":\"V\",\"PortLabel\":\"vParallelAssembly\",\"Probing\":\"ON\"}}"
  Module16_outputs : SimscapeProbe  BoundBlock=2688  Variables="{\"iCell\":{\"Unit\":\"A\",\"PortLabel\":\"iCell\",\"Probing\":\"ON\"},\"numCyclesCell\":{\"Unit\":\"1\",\"PortLabel\":\"numCyclesCell\",\"Probing\":\"ON\"},\"socCell\":{\"Unit\":\"1\",\"PortLabel\":\"socCell\",\"Probing\":\"ON\"},\"socParallelAssembly\":{\"Unit\":\"1\",\"PortLabel\":\"socParallelAssembly\",\"Probing\":\"ON\"},\"temperatureCell\":{\"Unit\":\"K\",\"PortLabel\":\"temperatureCell\",\"Probing\":\"ON\"},\"vCell\":{\"Unit\":\"V\",\"PortLabel\":\"vCell\",\"Probing\":\"ON\"},\"vParallelAssembly\":{\"Unit\":\"V\",\"PortLabel\":\"vParallelAssembly\",\"Probing\":\"ON\"}}"
  Module17_outputs : SimscapeProbe  BoundBlock=2690  Variables="{\"iCell\":{\"Unit\":\"A\",\"PortLabel\":\"iCell\",\"Probing\":\"ON\"},\"numCyclesCell\":{\"Unit\":\"1\",\"PortLabel\":\"numCyclesCell\",\"Probing\":\"ON\"},\"socCell\":{\"Unit\":\"1\",\"PortLabel\":\"socCell\",\"Probing\":\"ON\"},\"socParallelAssembly\":{\"Unit\":\"1\",\"PortLabel\":\"socParallelAssembly\",\"Probing\":\"ON\"},\"temperatureCell\":{\"Unit\":\"K\",\"PortLabel\":\"temperatureCell\",\"Probing\":\"ON\"},\"vCell\":{\"Unit\":\"V\",\"PortLabel\":\"vCell\",\"Probing\":\"ON\"},\"vParallelAssembly\":{\"Unit\":\"V\",\"PortLabel\":\"vParallelAssembly\",\"Probing\":\"ON\"}}"
  Module18_outputs : SimscapeProbe  BoundBlock=2692  Variables="{\"iCell\":{\"Unit\":\"A\",\"PortLabel\":\"iCell\",\"Probing\":\"ON\"},\"numCyclesCell\":{\"Unit\":\"1\",\"PortLabel\":\"numCyclesCell\",\"Probing\":\"ON\"},\"socCell\":{\"Unit\":\"1\",\"PortLabel\":\"socCell\",\"Probing\":\"ON\"},\"socParallelAssembly\":{\"Unit\":\"1\",\"PortLabel\":\"socParallelAssembly\",\"Probing\":\"ON\"},\"temperatureCell\":{\"Unit\":\"K\",\"PortLabel\":\"temperatureCell\",\"Probing\":\"ON\"},\"vCell\":{\"Unit\":\"V\",\"PortLabel\":\"vCell\",\"Probing\":\"ON\"},\"vParallelAssembly\":{\"Unit\":\"V\",\"PortLabel\":\"vParallelAssembly\",\"Probing\":\"ON\"}}"
  Module19_outputs : SimscapeProbe  BoundBlock=2694  Variables="{\"iCell\":{\"Unit\":\"A\",\"PortLabel\":\"iCell\",\"Probing\":\"ON\"},\"numCyclesCell\":{\"Unit\":\"1\",\"PortLabel\":\"numCyclesCell\",\"Probing\":\"ON\"},\"socCell\":{\"Unit\":\"1\",\"PortLabel\":\"socCell\",\"Probing\":\"ON\"},\"socParallelAssembly\":{\"Unit\":\"1\",\"PortLabel\":\"socParallelAssembly\",\"Probing\":\"ON\"},\"temperatureCell\":{\"Unit\":\"K\",\"PortLabel\":\"temperatureCell\",\"Probing\":\"ON\"},\"vCell\":{\"Unit\":\"V\",\"PortLabel\":\"vCell\",\"Probing\":\"ON\"},\"vParallelAssembly\":{\"Unit\":\"V\",\"PortLabel\":\"vParallelAssembly\",\"Probing\":\"ON\"}}"
  Module20_outputs : SimscapeProbe  BoundBlock=2696  Variables="{\"iCell\":{\"Unit\":\"A\",\"PortLabel\":\"iCell\",\"Probing\":\"ON\"},\"numCyclesCell\":{\"Unit\":\"1\",\"PortLabel\":\"numCyclesCell\",\"Probing\":\"ON\"},\"socCell\":{\"Unit\":\"1\",\"PortLabel\":\"socCell\",\"Probing\":\"ON\"},\"socParallelAssembly\":{\"Unit\":\"1\",\"PortLabel\":\"socParallelAssembly\",\"Probing\":\"ON\"},\"temperatureCell\":{\"Unit\":\"K\",\"PortLabel\":\"temperatureCell\",\"Probing\":\"ON\"},\"vCell\":{\"Unit\":\"V\",\"PortLabel\":\"vCell\",\"Probing\":\"ON\"},\"vParallelAssembly\":{\"Unit\":\"V\",\"PortLabel\":\"vParallelAssembly\",\"Probing\":\"ON\"}}"
  Module21_outputs : SimscapeProbe  BoundBlock=2698  Variables="{\"iCell\":{\"Unit\":\"A\",\"PortLabel\":\"iCell\",\"Probing\":\"ON\"},\"numCyclesCell\":{\"Unit\":\"1\",\"PortLabel\":\"numCyclesCell\",\"Probing\":\"ON\"},\"socCell\":{\"Unit\":\"1\",\"PortLabel\":\"socCell\",\"Probing\":\"ON\"},\"socParallelAssembly\":{\"Unit\":\"1\",\"PortLabel\":\"socParallelAssembly\",\"Probing\":\"ON\"},\"temperatureCell\":{\"Unit\":\"K\",\"PortLabel\":\"temperatureCell\",\"Probing\":\"ON\"},\"vCell\":{\"Unit\":\"V\",\"PortLabel\":\"vCell\",\"Probing\":\"ON\"},\"vParallelAssembly\":{\"Unit\":\"V\",\"PortLabel\":\"vParallelAssembly\",\"Probing\":\"ON\"}}"
  Module22_outputs : SimscapeProbe  BoundBlock=2700  Variables="{\"iCell\":{\"Unit\":\"A\",\"PortLabel\":\"iCell\",\"Probing\":\"ON\"},\"numCyclesCell\":{\"Unit\":\"1\",\"PortLabel\":\"numCyclesCell\",\"Probing\":\"ON\"},\"socCell\":{\"Unit\":\"1\",\"PortLabel\":\"socCell\",\"Probing\":\"ON\"},\"socParallelAssembly\":{\"Unit\":\"1\",\"PortLabel\":\"socParallelAssembly\",\"Probing\":\"ON\"},\"temperatureCell\":{\"Unit\":\"K\",\"PortLabel\":\"temperatureCell\",\"Probing\":\"ON\"},\"vCell\":{\"Unit\":\"V\",\"PortLabel\":\"vCell\",\"Probing\":\"ON\"},\"vParallelAssembly\":{\"Unit\":\"V\",\"PortLabel\":\"vParallelAssembly\",\"Probing\":\"ON\"}}"
  Module23_outputs : SimscapeProbe  BoundBlock=2702  Variables="{\"iCell\":{\"Unit\":\"A\",\"PortLabel\":\"iCell\",\"Probing\":\"ON\"},\"numCyclesCell\":{\"Unit\":\"1\",\"PortLabel\":\"numCyclesCell\",\"Probing\":\"ON\"},\"socCell\":{\"Unit\":\"1\",\"PortLabel\":\"socCell\",\"Probing\":\"ON\"},\"socParallelAssembly\":{\"Unit\":\"1\",\"PortLabel\":\"socParallelAssembly\",\"Probing\":\"ON\"},\"temperatureCell\":{\"Unit\":\"K\",\"PortLabel\":\"temperatureCell\",\"Probing\":\"ON\"},\"vCell\":{\"Unit\":\"V\",\"PortLabel\":\"vCell\",\"Probing\":\"ON\"},\"vParallelAssembly\":{\"Unit\":\"V\",\"PortLabel\":\"vParallelAssembly\",\"Probing\":\"ON\"}}"
  Module_1_1 : BatteryPack_v2_lib/Modules/ModuleType1  SOC_vecCell=[0, .1, .25, .5, .75, .9, 1]  T_vecCell=[278, 293, 313] K  V0_matCell=[3.49, 3.5, 3.51; 3.55, 3.57, 3.56; 3.62, 3.63, 3.64; 3.71, 3.71, 3.72; 3.91, 3.93, 3.94; 4.07, 4.08, 4.08; 4.19, 4.19, 4.19] V  V_rangeCell=[0, inf] V  R0_matCell=[.0117, .0085, .009; .011, .0085, .009; .0114, .0087, .0092; .0107, .0082, .0088; .0107, .0083, .0091; .0113, .0085, .0089; .0116, .0085, .0089] Ohm  AHCell=27 A*hr  extrapolation_optionCell=simscape.enum.extrapolation.nearest  N0Cell=100  dV0Cell=0  dR0Cell=0  dAHCell=0  thermal_massCell=100 J/K  AmbientResistance=25 K/W  P=1  S=1  iCell_specify=off  iCell_priority=None  iCell=0 A  iCell_nominal_specify=off  iCell_nominal_value=1  iCell_nominal_unit=A  vCell_specify=off  vCell_priority=None  vCell=0 V  vCell_nominal_specify=off  vCell_nominal_value=1  vCell_nominal_unit=V  socCell_specify=off  socCell_priority=High  socCell=1  socCell_nominal_specify=off  socCell_nominal_value=1  socCell_nominal_unit=1  numCyclesCell_specify=off  numCyclesCell_priority=High  numCyclesCell=0  numCyclesCell_nominal_specify=off  numCyclesCell_nominal_value=1  numCyclesCell_nominal_unit=1  temperatureCell_specify=off  temperatureCell_priority=High  temperatureCell=298.15 K  temperatureCell_nominal_specify=off  temperatureCell_nominal_value=1  temperatureCell_nominal_unit=K  vParallelAssembly_specify=off  vParallelAssembly_priority=None  vParallelAssembly=0 V  vParallelAssembly_nominal_specify=off  vParallelAssembly_nominal_value=1  vParallelAssembly_nominal_unit=V  socParallelAssembly_specify=off  socParallelAssembly_priority=None  socParallelAssembly=1  socParallelAssembly_nominal_specify=off  socParallelAssembly_nominal_value=1  socParallelAssembly_nominal_unit=1
      settings: InternalSimscapePortConfiguration="{\"Bottom\":[{\"id\":\"n\",\"label\":\"-\",\"type\":\"foundation.electrical.electrical\"}],\"Left\":[{\"id\":\"AmbH\",\"label\":\"AmbH\",\"type\":\"foundation.thermal.thermal\"}],\"Right\":[],\"Top\":[{\"id\":\"p\",\"label\":\"+\",\"type\":\"foundation.electrical.electrical\"}]}"
  Module_1_1_outputs : SimscapeProbe  BoundBlock=2704  Variables="{\"iCell\":{\"Unit\":\"A\",\"PortLabel\":\"iCell\",\"Probing\":\"ON\"},\"numCyclesCell\":{\"Unit\":\"1\",\"PortLabel\":\"numCyclesCell\",\"Probing\":\"ON\"},\"socCell\":{\"Unit\":\"1\",\"PortLabel\":\"socCell\",\"Probing\":\"ON\"},\"socParallelAssembly\":{\"Unit\":\"1\",\"PortLabel\":\"socParallelAssembly\",\"Probing\":\"ON\"},\"temperatureCell\":{\"Unit\":\"K\",\"PortLabel\":\"temperatureCell\",\"Probing\":\"ON\"},\"vCell\":{\"Unit\":\"V\",\"PortLabel\":\"vCell\",\"Probing\":\"ON\"},\"vParallelAssembly\":{\"Unit\":\"V\",\"PortLabel\":\"vParallelAssembly\",\"Probing\":\"ON\"}}"
  iCellMux : Mux  Inputs=23
  numCyclesCellMux : Mux  Inputs=23
  socCellMux : Mux  Inputs=23
  socParallelAssemblyMux : Mux  Inputs=23
  temperatureCellMux : Mux  Inputs=23
  vCellMux : Mux  Inputs=23
  vParallelAssemblyMux : Mux  Inputs=23
  + : PMIOPort  Side=Left
  - : PMIOPort  Port=2  Side=Right
  AmbH : PMIOPort  Port=3  Side=Right  ConnectionType=Connection: foundation.thermal.thermal
  iCell : Outport
  numCyclesCell : Outport  Port=2
  socCell : Outport  Port=3
  socParallelAssembly : Outport  Port=4
  temperatureCell : Outport  Port=5
  vCell : Outport  Port=6
  vParallelAssembly : Outport  Port=7
  wires:
  [vParallelAssembly23] -> vParallelAssemblyMux/23
  Module23_outputs/7 -> [vParallelAssembly23]
  [vCell23] -> vCellMux/23
  Module23_outputs/6 -> [vCell23]
  [temperatureCell23] -> temperatureCellMux/23
  Module23_outputs/5 -> [temperatureCell23]
  [socParallelAssembly23] -> socParallelAssemblyMux/23
  Module23_outputs/4 -> [socParallelAssembly23]
  [socCell23] -> socCellMux/23
  Module23_outputs/3 -> [socCell23]
  [numCyclesCell23] -> numCyclesCellMux/23
  Module23_outputs/2 -> [numCyclesCell23]
  [iCell23] -> iCellMux/23
  Module23_outputs/1 -> [iCell23]
  [vParallelAssembly22] -> vParallelAssemblyMux/22
  Module22_outputs/7 -> [vParallelAssembly22]
  [vCell22] -> vCellMux/22
  Module22_outputs/6 -> [vCell22]
  [temperatureCell22] -> temperatureCellMux/22
  Module22_outputs/5 -> [temperatureCell22]
  [socParallelAssembly22] -> socParallelAssemblyMux/22
  Module22_outputs/4 -> [socParallelAssembly22]
  [socCell22] -> socCellMux/22
  Module22_outputs/3 -> [socCell22]
  [numCyclesCell22] -> numCyclesCellMux/22
  Module22_outputs/2 -> [numCyclesCell22]
  [iCell22] -> iCellMux/22
  Module22_outputs/1 -> [iCell22]
  [vParallelAssembly21] -> vParallelAssemblyMux/21
  Module21_outputs/7 -> [vParallelAssembly21]
  [vCell21] -> vCellMux/21
  Module21_outputs/6 -> [vCell21]
  [temperatureCell21] -> temperatureCellMux/21
  Module21_outputs/5 -> [temperatureCell21]
  [socParallelAssembly21] -> socParallelAssemblyMux/21
  Module21_outputs/4 -> [socParallelAssembly21]
  [socCell21] -> socCellMux/21
  Module21_outputs/3 -> [socCell21]
  [numCyclesCell21] -> numCyclesCellMux/21
  Module21_outputs/2 -> [numCyclesCell21]
  [iCell21] -> iCellMux/21
  Module21_outputs/1 -> [iCell21]
  [vParallelAssembly20] -> vParallelAssemblyMux/20
  Module20_outputs/7 -> [vParallelAssembly20]
  [vCell20] -> vCellMux/20
  Module20_outputs/6 -> [vCell20]
  [temperatureCell20] -> temperatureCellMux/20
  Module20_outputs/5 -> [temperatureCell20]
  [socParallelAssembly20] -> socParallelAssemblyMux/20
  Module20_outputs/4 -> [socParallelAssembly20]
  [socCell20] -> socCellMux/20
  Module20_outputs/3 -> [socCell20]
  [numCyclesCell20] -> numCyclesCellMux/20
  Module20_outputs/2 -> [numCyclesCell20]
  [iCell20] -> iCellMux/20
  Module20_outputs/1 -> [iCell20]
  [vParallelAssembly19] -> vParallelAssemblyMux/19
  Module19_outputs/7 -> [vParallelAssembly19]
  [vCell19] -> vCellMux/19
  Module19_outputs/6 -> [vCell19]
  [temperatureCell19] -> temperatureCellMux/19
  Module19_outputs/5 -> [temperatureCell19]
  [socParallelAssembly19] -> socParallelAssemblyMux/19
  Module19_outputs/4 -> [socParallelAssembly19]
  [socCell19] -> socCellMux/19
  Module19_outputs/3 -> [socCell19]
  [numCyclesCell19] -> numCyclesCellMux/19
  Module19_outputs/2 -> [numCyclesCell19]
  [iCell19] -> iCellMux/19
  Module19_outputs/1 -> [iCell19]
  [vParallelAssembly18] -> vParallelAssemblyMux/18
  Module18_outputs/7 -> [vParallelAssembly18]
  [vCell18] -> vCellMux/18
  Module18_outputs/6 -> [vCell18]
  [temperatureCell18] -> temperatureCellMux/18
  Module18_outputs/5 -> [temperatureCell18]
  [socParallelAssembly18] -> socParallelAssemblyMux/18
  Module18_outputs/4 -> [socParallelAssembly18]
  [socCell18] -> socCellMux/18
  Module18_outputs/3 -> [socCell18]
  [numCyclesCell18] -> numCyclesCellMux/18
  Module18_outputs/2 -> [numCyclesCell18]
  [iCell18] -> iCellMux/18
  Module18_outputs/1 -> [iCell18]
  [vParallelAssembly17] -> vParallelAssemblyMux/17
  Module17_outputs/7 -> [vParallelAssembly17]
  [vCell17] -> vCellMux/17
  Module17_outputs/6 -> [vCell17]
  [temperatureCell17] -> temperatureCellMux/17
  Module17_outputs/5 -> [temperatureCell17]
  [socParallelAssembly17] -> socParallelAssemblyMux/17
  Module17_outputs/4 -> [socParallelAssembly17]
  [socCell17] -> socCellMux/17
  Module17_outputs/3 -> [socCell17]
  [numCyclesCell17] -> numCyclesCellMux/17
  Module17_outputs/2 -> [numCyclesCell17]
  [iCell17] -> iCellMux/17
  Module17_outputs/1 -> [iCell17]
  [vParallelAssembly16] -> vParallelAssemblyMux/16
  Module16_outputs/7 -> [vParallelAssembly16]
  [vCell16] -> vCellMux/16
  Module16_outputs/6 -> [vCell16]
  [temperatureCell16] -> temperatureCellMux/16
  Module16_outputs/5 -> [temperatureCell16]
  [socParallelAssembly16] -> socParallelAssemblyMux/16
  Module16_outputs/4 -> [socParallelAssembly16]
  [socCell16] -> socCellMux/16
  Module16_outputs/3 -> [socCell16]
  [numCyclesCell16] -> numCyclesCellMux/16
  Module16_outputs/2 -> [numCyclesCell16]
  [iCell16] -> iCellMux/16
  Module16_outputs/1 -> [iCell16]
  [vParallelAssembly15] -> vParallelAssemblyMux/15
  Module15_outputs/7 -> [vParallelAssembly15]
  [vCell15] -> vCellMux/15
  Module15_outputs/6 -> [vCell15]
  [temperatureCell15] -> temperatureCellMux/15
  Module15_outputs/5 -> [temperatureCell15]
  [socParallelAssembly15] -> socParallelAssemblyMux/15
  Module15_outputs/4 -> [socParallelAssembly15]
  [socCell15] -> socCellMux/15
  Module15_outputs/3 -> [socCell15]
  [numCyclesCell15] -> numCyclesCellMux/15
  Module15_outputs/2 -> [numCyclesCell15]
  [iCell15] -> iCellMux/15
  Module15_outputs/1 -> [iCell15]
  [vParallelAssembly14] -> vParallelAssemblyMux/14
  Module14_outputs/7 -> [vParallelAssembly14]
  [vCell14] -> vCellMux/14
  Module14_outputs/6 -> [vCell14]
  [temperatureCell14] -> temperatureCellMux/14
  Module14_outputs/5 -> [temperatureCell14]
  [socParallelAssembly14] -> socParallelAssemblyMux/14
  Module14_outputs/4 -> [socParallelAssembly14]
  [socCell14] -> socCellMux/14
  Module14_outputs/3 -> [socCell14]
  [numCyclesCell14] -> numCyclesCellMux/14
  Module14_outputs/2 -> [numCyclesCell14]
  [iCell14] -> iCellMux/14
  Module14_outputs/1 -> [iCell14]
  [vParallelAssembly13] -> vParallelAssemblyMux/13
  Module13_outputs/7 -> [vParallelAssembly13]
  [vCell13] -> vCellMux/13
  Module13_outputs/6 -> [vCell13]
  [temperatureCell13] -> temperatureCellMux/13
  Module13_outputs/5 -> [temperatureCell13]
  [socParallelAssembly13] -> socParallelAssemblyMux/13
  Module13_outputs/4 -> [socParallelAssembly13]
  [socCell13] -> socCellMux/13
  Module13_outputs/3 -> [socCell13]
  [numCyclesCell13] -> numCyclesCellMux/13
  Module13_outputs/2 -> [numCyclesCell13]
  [iCell13] -> iCellMux/13
  Module13_outputs/1 -> [iCell13]
  [vParallelAssembly12] -> vParallelAssemblyMux/12
  Module12_outputs/7 -> [vParallelAssembly12]
  [vCell12] -> vCellMux/12
  Module12_outputs/6 -> [vCell12]
  [temperatureCell12] -> temperatureCellMux/12
  Module12_outputs/5 -> [temperatureCell12]
  [socParallelAssembly12] -> socParallelAssemblyMux/12
  Module12_outputs/4 -> [socParallelAssembly12]
  [socCell12] -> socCellMux/12
  Module12_outputs/3 -> [socCell12]
  [numCyclesCell12] -> numCyclesCellMux/12
  Module12_outputs/2 -> [numCyclesCell12]
  [iCell12] -> iCellMux/12
  Module12_outputs/1 -> [iCell12]
  [vParallelAssembly11] -> vParallelAssemblyMux/11
  Module11_outputs/7 -> [vParallelAssembly11]
  [vCell11] -> vCellMux/11
  Module11_outputs/6 -> [vCell11]
  [temperatureCell11] -> temperatureCellMux/11
  Module11_outputs/5 -> [temperatureCell11]
  [socParallelAssembly11] -> socParallelAssemblyMux/11
  Module11_outputs/4 -> [socParallelAssembly11]
  [socCell11] -> socCellMux/11
  Module11_outputs/3 -> [socCell11]
  [numCyclesCell11] -> numCyclesCellMux/11
  Module11_outputs/2 -> [numCyclesCell11]
  [iCell11] -> iCellMux/11
  Module11_outputs/1 -> [iCell11]
  [vParallelAssembly10] -> vParallelAssemblyMux/10
  Module10_outputs/7 -> [vParallelAssembly10]
  [vCell10] -> vCellMux/10
  Module10_outputs/6 -> [vCell10]
  [temperatureCell10] -> temperatureCellMux/10
  Module10_outputs/5 -> [temperatureCell10]
  [socParallelAssembly10] -> socParallelAssemblyMux/10
  Module10_outputs/4 -> [socParallelAssembly10]
  [socCell10] -> socCellMux/10
  Module10_outputs/3 -> [socCell10]
  [numCyclesCell10] -> numCyclesCellMux/10
  Module10_outputs/2 -> [numCyclesCell10]
  [iCell10] -> iCellMux/10
  Module10_outputs/1 -> [iCell10]
  [vParallelAssembly9] -> vParallelAssemblyMux/9
  Module09_outputs/7 -> [vParallelAssembly9]
  [vCell9] -> vCellMux/9
  Module09_outputs/6 -> [vCell9]
  [temperatureCell9] -> temperatureCellMux/9
  Module09_outputs/5 -> [temperatureCell9]
  [socParallelAssembly9] -> socParallelAssemblyMux/9
  Module09_outputs/4 -> [socParallelAssembly9]
  [socCell9] -> socCellMux/9
  Module09_outputs/3 -> [socCell9]
  [numCyclesCell9] -> numCyclesCellMux/9
  Module09_outputs/2 -> [numCyclesCell9]
  [iCell9] -> iCellMux/9
  Module09_outputs/1 -> [iCell9]
  [vParallelAssembly8] -> vParallelAssemblyMux/8
  Module08_outputs/7 -> [vParallelAssembly8]
  [vCell8] -> vCellMux/8
  Module08_outputs/6 -> [vCell8]
  [temperatureCell8] -> temperatureCellMux/8
  Module08_outputs/5 -> [temperatureCell8]
  [socParallelAssembly8] -> socParallelAssemblyMux/8
  Module08_outputs/4 -> [socParallelAssembly8]
  [socCell8] -> socCellMux/8
  Module08_outputs/3 -> [socCell8]
  [numCyclesCell8] -> numCyclesCellMux/8
  Module08_outputs/2 -> [numCyclesCell8]
  [iCell8] -> iCellMux/8
  Module08_outputs/1 -> [iCell8]
  [vParallelAssembly7] -> vParallelAssemblyMux/7
  Module07_outputs/7 -> [vParallelAssembly7]
  [vCell7] -> vCellMux/7
  Module07_outputs/6 -> [vCell7]
  [temperatureCell7] -> temperatureCellMux/7
  Module07_outputs/5 -> [temperatureCell7]
  [socParallelAssembly7] -> socParallelAssemblyMux/7
  Module07_outputs/4 -> [socParallelAssembly7]
  [socCell7] -> socCellMux/7
  Module07_outputs/3 -> [socCell7]
  [numCyclesCell7] -> numCyclesCellMux/7
  Module07_outputs/2 -> [numCyclesCell7]
  [iCell7] -> iCellMux/7
  Module07_outputs/1 -> [iCell7]
  [vParallelAssembly6] -> vParallelAssemblyMux/6
  Module06_outputs/7 -> [vParallelAssembly6]
  [vCell6] -> vCellMux/6
  Module06_outputs/6 -> [vCell6]
  [temperatureCell6] -> temperatureCellMux/6
  Module06_outputs/5 -> [temperatureCell6]
  [socParallelAssembly6] -> socParallelAssemblyMux/6
  Module06_outputs/4 -> [socParallelAssembly6]
  [socCell6] -> socCellMux/6
  Module06_outputs/3 -> [socCell6]
  [numCyclesCell6] -> numCyclesCellMux/6
  Module06_outputs/2 -> [numCyclesCell6]
  [iCell6] -> iCellMux/6
  Module06_outputs/1 -> [iCell6]
  [vParallelAssembly5] -> vParallelAssemblyMux/5
  Module05_outputs/7 -> [vParallelAssembly5]
  [vCell5] -> vCellMux/5
  Module05_outputs/6 -> [vCell5]
  [temperatureCell5] -> temperatureCellMux/5
  Module05_outputs/5 -> [temperatureCell5]
  [socParallelAssembly5] -> socParallelAssemblyMux/5
  Module05_outputs/4 -> [socParallelAssembly5]
  [socCell5] -> socCellMux/5
  Module05_outputs/3 -> [socCell5]
  [numCyclesCell5] -> numCyclesCellMux/5
  Module05_outputs/2 -> [numCyclesCell5]
  [iCell5] -> iCellMux/5
  Module05_outputs/1 -> [iCell5]
  [vParallelAssembly4] -> vParallelAssemblyMux/4
  Module04_outputs/7 -> [vParallelAssembly4]
  [vCell4] -> vCellMux/4
  Module04_outputs/6 -> [vCell4]
  [temperatureCell4] -> temperatureCellMux/4
  Module04_outputs/5 -> [temperatureCell4]
  [socParallelAssembly4] -> socParallelAssemblyMux/4
  Module04_outputs/4 -> [socParallelAssembly4]
  [socCell4] -> socCellMux/4
  Module04_outputs/3 -> [socCell4]
  [numCyclesCell4] -> numCyclesCellMux/4
  Module04_outputs/2 -> [numCyclesCell4]
  [iCell4] -> iCellMux/4
  Module04_outputs/1 -> [iCell4]
  [vParallelAssembly3] -> vParallelAssemblyMux/3
  Module03_outputs/7 -> [vParallelAssembly3]
  [vCell3] -> vCellMux/3
  Module03_outputs/6 -> [vCell3]
  [temperatureCell3] -> temperatureCellMux/3
  Module03_outputs/5 -> [temperatureCell3]
  [socParallelAssembly3] -> socParallelAssemblyMux/3
  Module03_outputs/4 -> [socParallelAssembly3]
  [socCell3] -> socCellMux/3
  Module03_outputs/3 -> [socCell3]
  [numCyclesCell3] -> numCyclesCellMux/3
  Module03_outputs/2 -> [numCyclesCell3]
  [iCell3] -> iCellMux/3
  Module03_outputs/1 -> [iCell3]
  [vParallelAssembly2] -> vParallelAssemblyMux/2
  Module02_outputs/7 -> [vParallelAssembly2]
  [vCell2] -> vCellMux/2
  Module02_outputs/6 -> [vCell2]
  [temperatureCell2] -> temperatureCellMux/2
  Module02_outputs/5 -> [temperatureCell2]
  [socParallelAssembly2] -> socParallelAssemblyMux/2
  Module02_outputs/4 -> [socParallelAssembly2]
  [socCell2] -> socCellMux/2
  Module02_outputs/3 -> [socCell2]
  [numCyclesCell2] -> numCyclesCellMux/2
  Module02_outputs/2 -> [numCyclesCell2]
  [iCell2] -> iCellMux/2
  Module02_outputs/1 -> [iCell2]
  [vParallelAssembly1] -> vParallelAssemblyMux/1
  vParallelAssemblyMux/1 -> vParallelAssembly/1
  Module_1_1_outputs/7 -> [vParallelAssembly1]
  [vCell1] -> vCellMux/1
  vCellMux/1 -> vCell/1
  Module_1_1_outputs/6 -> [vCell1]
  [temperatureCell1] -> temperatureCellMux/1
  temperatureCellMux/1 -> temperatureCell/1
  Module_1_1_outputs/5 -> [temperatureCell1]
  [socParallelAssembly1] -> socParallelAssemblyMux/1
  socParallelAssemblyMux/1 -> socParallelAssembly/1
  Module_1_1_outputs/4 -> [socParallelAssembly1]
  [socCell1] -> socCellMux/1
  socCellMux/1 -> socCell/1
  Module_1_1_outputs/3 -> [socCell1]
  [numCyclesCell1] -> numCyclesCellMux/1
  numCyclesCellMux/1 -> numCyclesCell/1
  Module_1_1_outputs/2 -> [numCyclesCell1]
  [iCell1] -> iCellMux/1
  iCellMux/1 -> iCell/1
  Module_1_1_outputs/1 -> [iCell1]
  connections:
  AmbH_To_23/LConn1 -- Module23/LConn1
  AmbH_To_22/LConn1 -- Module22/LConn1
  AmbH_To_21/LConn1 -- Module21/LConn1
  AmbH_To_20/LConn1 -- Module20/LConn1
  AmbH_To_19/LConn1 -- Module19/LConn1
  AmbH_To_18/LConn1 -- Module18/LConn1
  AmbH_To_17/LConn1 -- Module17/LConn1
  AmbH_To_16/LConn1 -- Module16/LConn1
  AmbH_To_15/LConn1 -- Module15/LConn1
  AmbH_To_14/LConn1 -- Module14/LConn1
  AmbH_To_13/LConn1 -- Module13/LConn1
  AmbH_To_12/LConn1 -- Module12/LConn1
  AmbH_To_11/LConn1 -- Module11/LConn1
  AmbH_To_10/LConn1 -- Module10/LConn1
  AmbH_To_9/LConn1 -- Module09/LConn1
  AmbH_To_8/LConn1 -- Module08/LConn1
  AmbH_To_7/LConn1 -- Module07/LConn1
  AmbH_To_6/LConn1 -- Module06/LConn1
  AmbH_To_5/LConn1 -- Module05/LConn1
  AmbH_To_4/LConn1 -- Module04/LConn1
  AmbH_To_3/LConn1 -- Module03/LConn1
  AmbH_To_2/LConn1 -- Module02/LConn1
  AmbH_From_23/LConn1 -- AmbH/RConn1 -- AmbH_From_22/LConn1 -- AmbH_From_21/LConn1 -- AmbH_From_20/LConn1 -- AmbH_From_19/LConn1 -- AmbH_From_18/LConn1 -- AmbH_From_17/LConn1 -- AmbH_From_16/LConn1 -- AmbH_From_15/LConn1 -- AmbH_From_14/LConn1 -- AmbH_From_13/LConn1 -- AmbH_From_12/LConn1 -- AmbH_From_11/LConn1 -- AmbH_From_10/LConn1 -- AmbH_From_9/LConn1 -- AmbH_From_8/LConn1 -- AmbH_From_7/LConn1 -- AmbH_From_6/LConn1 -- AmbH_From_5/LConn1 -- AmbH_From_4/LConn1 -- AmbH_From_3/LConn1 -- AmbH_From_2/LConn1 -- AmbH_From_1/LConn1
  AmbH_To_1/LConn1 -- Module_1_1/LConn1
  Module23/RConn1 -- -/RConn1
  Module_1_1/LConn2 -- +/RConn1
  Module23/LConn2 -- Module22/RConn1
  Module22/LConn2 -- Module21/RConn1
  Module21/LConn2 -- Module20/RConn1
  Module20/LConn2 -- Module19/RConn1
  Module19/LConn2 -- Module18/RConn1
  Module18/LConn2 -- Module17/RConn1
  Module17/LConn2 -- Module16/RConn1
  Module16/LConn2 -- Module15/RConn1
  Module15/LConn2 -- Module14/RConn1
  Module14/LConn2 -- Module13/RConn1
  Module13/LConn2 -- Module12/RConn1
  Module12/LConn2 -- Module11/RConn1
  Module11/LConn2 -- Module10/RConn1
  Module10/LConn2 -- Module09/RConn1
  Module09/LConn2 -- Module08/RConn1
  Module08/LConn2 -- Module07/RConn1
  Module07/LConn2 -- Module06/RConn1
  Module06/LConn2 -- Module05/RConn1
  Module05/LConn2 -- Module04/RConn1
  Module04/LConn2 -- Module03/RConn1
  Module03/LConn2 -- Module02/RConn1
  Module02/LConn2 -- Module_1_1/RConn1
